simulink model "sim_topic3"  (R2023b)
settings: Solver=VariableStepAuto  StartTime=0.0  StopTime=N  RelTol=1e-3
undefined symbols (not defined in the file): Ad, Bd, Cd, Dd, T, xd0
settings Model: Creator=user  LastModifiedBy=user

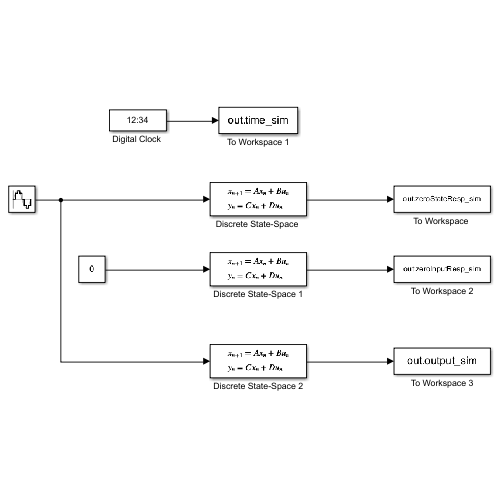
[thumbnail: Simulink's stored preview of the top-level diagram]
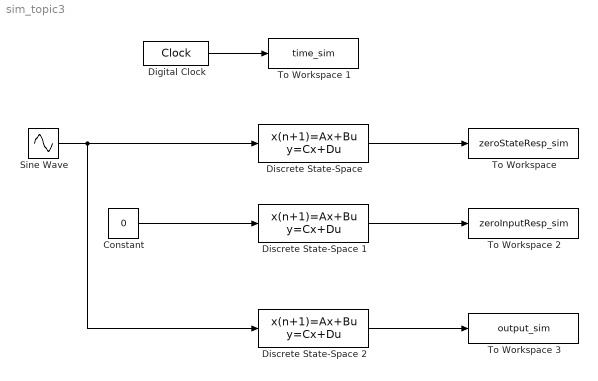
== system sim_topic3 ==
  Constant : Constant  Value=0  SampleTime=T
  "Digital Clock " : DigitalClock  SampleTime=T
  "Discrete State-Space " : DiscreteStateSpace  A=Ad  B=Bd  C=Cd  D=Dd  SampleTime=T
  Discrete State-Space 1 : DiscreteStateSpace  A=Ad  B=Bd  C=Cd  D=Dd  InitialCondition=xd0  SampleTime=T
  Discrete State-Space 2 : DiscreteStateSpace  A=Ad  B=Bd  C=Cd  D=Dd  InitialCondition=xd0  SampleTime=T
  Sine Wave : Sin  Amplitude=0.1  Frequency=0.5  SampleTime=T
  "To Workspace " : ToWorkspace  VariableName=zeroStateResp_sim  SampleTime=T
  To Workspace 1 : ToWorkspace  VariableName=time_sim  SampleTime=-1
  To Workspace 2 : ToWorkspace  VariableName=zeroInputResp_sim  SampleTime=T
  To Workspace 3 : ToWorkspace  VariableName=output_sim  SampleTime=T
  wires:
  "Discrete State-Space "/1 -> "To Workspace "/1
  "Digital Clock "/1 -> To Workspace 1/1
  Discrete State-Space 1/1 -> To Workspace 2/1
  Constant/1 -> Discrete State-Space 1/1
  Discrete State-Space 2/1 -> To Workspace 3/1
  Sine Wave/1 -> Discrete State-Space 2/1, "Discrete State-Space "/1
